simulink model "untitled1"  (R2023b)
settings: Solver=VariableStepAuto  StartTime=0.0  StopTime=10.0  RelTol=1e-3
undefined symbols (not defined in the file or in its folder): magnitude
libraries: dspfdesign x3
settings Model: Creator=mrabd  LastModifiedBy=mrabd

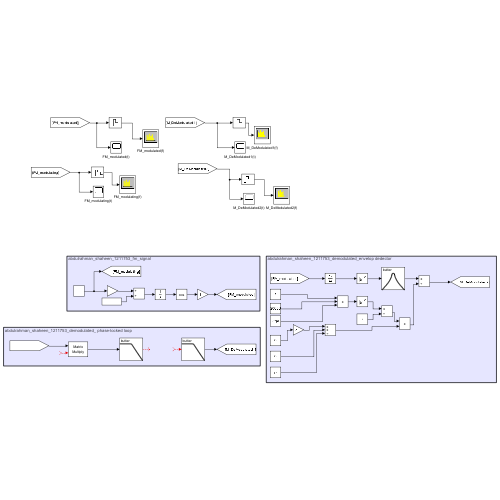
[thumbnail: Simulink's stored preview of the top-level diagram]
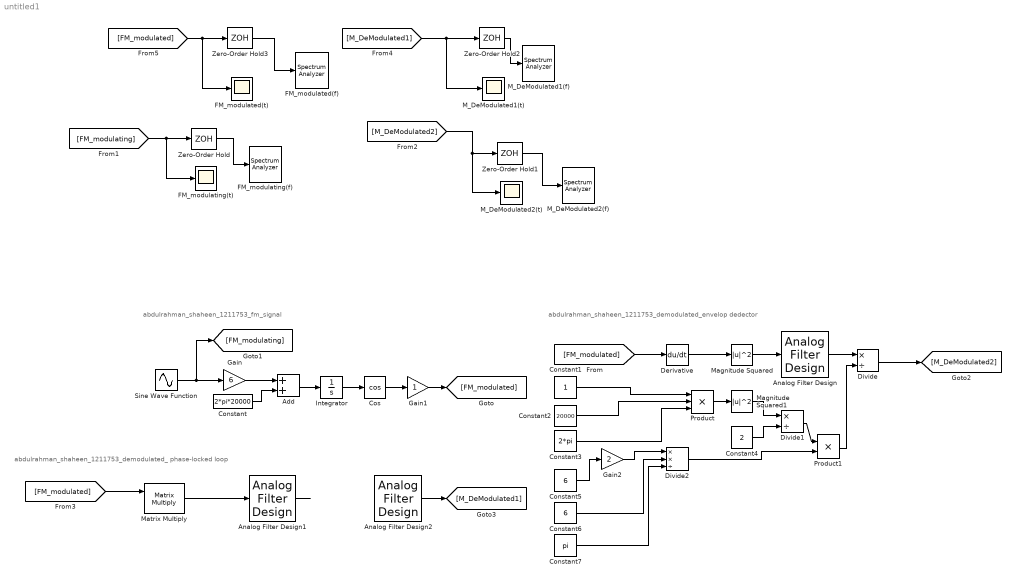
== system untitled1 ==
  note: abdulrahman_shaheen_1211753_demodulated_ phase-locked loop
  note: abdulrahman_shaheen_1211753_demodulated_envelop dedector
  note: abdulrahman_shaheen_1211753_fm_signal
  Add : Sum
  Analog Filter Design : dspfdesign/Analog Filter Design  method=Butterworth  filttype=Bandpass  N=8  Wlo=16500  Whi=23500  Rp=2  Rs=40
  Analog Filter Design1 : dspfdesign/Analog Filter Design  method=Butterworth  filttype=Lowpass  N=8  Wlo=30  Whi=80  Rp=2  Rs=40
  Analog Filter Design2 : dspfdesign/Analog Filter Design  method=Butterworth  filttype=Lowpass  N=8  Wlo=30  Whi=80  Rp=2  Rs=40
  Constant : Constant  Value=2*pi*20000
  Constant1 : Constant
  Constant2 : Constant  Value=20000
  Constant3 : Constant  Value=2*pi
  Constant4 : Constant  Value=2
  Constant5 : Constant  Value=6
  Constant6 : Constant  Value=6
  Constant7 : Constant  Value=pi
  Cos : Trigonometry  Operator=cos
  Derivative : Derivative
  Divide : Product  Inputs=*/
  Divide1 : Product  Inputs=*/
  Divide2 : Product  Inputs=**/
  FM_modulated(f) : SpectrumAnalyzer  WindowPosition=[2.000000,454.000000,766.000000,381.000000,]  ScopeFrameLocation=window  SampleRateSource=Property  SampleRate=44.1e3  PlotAsTwoSidedSpectrum=off  FrequencyScale=Log  FrequencySpan=Start and stop frequencies  StartFrequency=20  StopFrequency=20e3  YLimits=[-196.2865554,-59.04923233]
  FM_modulated(t) : Scope
  FM_modulating(f) : SpectrumAnalyzer  WindowPosition=[2.000000,48.000000,766.000000,374.000000,]  ScopeFrameLocation=window  SampleRateSource=Property  SampleRate=44.1e3  PlotAsTwoSidedSpectrum=off  FrequencyScale=Log  FrequencySpan=Start and stop frequencies  StartFrequency=20  StopFrequency=20e3  YLimits=[-255.26448155,-51.86972253]
  FM_modulating(t) : Scope
  Gain : Gain  Gain=6
  Gain1 : Gain
  Gain2 : Gain  Gain=2
  Integrator : Integrator
  M_DeModulated1(f) : SpectrumAnalyzer  WindowPosition=[368.000000,182.000000,800.000000,500.000000,]  Visible=on  ScopeFrameLocation=window  SampleRateSource=Property  SampleRate=44.1e3  PlotAsTwoSidedSpectrum=off  FrequencyScale=Log  FrequencySpan=Start and stop frequencies  StartFrequency=20  StopFrequency=20e3  YLimits=[-3603.44492261,-2802.67938425]
  M_DeModulated1(t) : Scope
  M_DeModulated2(f) : SpectrumAnalyzer  WindowPosition=[770.000000,42.000000,766.000000,793.000000,]  ScopeFrameLocation=window  SampleRateSource=Property  SampleRate=44.1e3  PlotAsTwoSidedSpectrum=off  FrequencyScale=Log  FrequencySpan=Start and stop frequencies  StartFrequency=20  StopFrequency=20e3  YLimits=[-197.56755721,-147.26404217]
  M_DeModulated2(t) : Scope
  Magnitude Squared : Math  Operator=magnitude^2
  Magnitude Squared1 : Math  Operator=magnitude^2
  Matrix Multiply : Product  Multiplication=Matrix(*)
  Product : Product  Inputs=3
  Product1 : Product
  Sine Wave Function : Sin  Frequency=1000  SampleTime=0
  Zero-Order Hold{,1..3} (4 alike) : ZeroOrderHold  SampleTime=-1
  wires:
  Integrator/1 -> Cos/1
  Gain/1 -> Add/1
  Gain1/1 -> [FM_modulated]
  Cos/1 -> Gain1/1
  Add/1 -> Integrator/1
  Constant/1 -> Add/2
  Sine Wave Function/1 -> [FM_modulating], Gain/1
  Magnitude Squared/1 -> Analog Filter Design/1
  Constant6/1 -> Divide2/2
  [FM_modulated] -> Derivative/1
  Divide/1 -> [M_DeModulated2]
  Analog Filter Design/1 -> Divide/1
  Constant2/1 -> Product/2
  Constant4/1 -> Divide1/2
  Derivative/1 -> Magnitude Squared/1
  Constant1/1 -> Product/1
  Constant5/1 -> Gain2/1
  Product1/1 -> Divide/2
  Divide1/1 -> Product1/1
  Magnitude Squared1/1 -> Divide1/1
  Product/1 -> Magnitude Squared1/1
  Constant7/1 -> Divide2/3
  Gain2/1 -> Divide2/1
  Divide2/1 -> Product1/2
  Constant3/1 -> Product/3
  ? -> Analog Filter Design2/1
  ? -> Matrix Multiply/2
  Analog Filter Design1/1 -> ?
  [FM_modulated] -> Matrix Multiply/1
  Analog Filter Design2/1 -> [M_DeModulated1]
  Matrix Multiply/1 -> Analog Filter Design1/1
  [FM_modulating] -> FM_modulating(t)/1, Zero-Order Hold/1
  Zero-Order Hold/1 -> FM_modulating(f)/1
  [M_DeModulated2] -> M_DeModulated2(t)/1, Zero-Order Hold1/1
  Zero-Order Hold1/1 -> M_DeModulated2(f)/1
  [M_DeModulated1] -> M_DeModulated1(t)/1, Zero-Order Hold2/1
  Zero-Order Hold2/1 -> M_DeModulated1(f)/1
  [FM_modulated] -> FM_modulated(t)/1, Zero-Order Hold3/1
  Zero-Order Hold3/1 -> FM_modulated(f)/1
